simulink model "traj_gene_data"  (R2018b)
settings: Solver=ode4  StartTime=0.0  StopTime=floor(cmd(end,1))  FixedStep=dt_solve  RelTol=1e-3
StopFcn:
  | for k=2:size(imu_delta,1)
  | imu_delta(k-1,2:7) = imu_delta(k,2:7)-imu_delta(k-1,2:7);
  | end
  | imu_delta(1:end-1,1) = imu_delta(2:end,1);
  | imu_delta(end,:) = [];
  | clearvars k
  | save([path,'/traj.mat'], 'traj_m','imu_rate','imu_delta');
values from neighbouring files (symbols this model uses):
  cmd = zeros(1,6)    [traj_design.m]
undefined symbols (not defined in the file or in its folder): data, Earth, Pv, WGS84
libraries: aerolibgravity2 x2, aerolibutil x2, sharedtransform x2, aerolib6dof2 x1, aerolibconvert2 x1
settings Model: Creator=longt  LastModifiedBy=longt
settings DataIOCC: SaveOutput=off  SignalLogging=off  DSMLogging=off  SaveTime=off

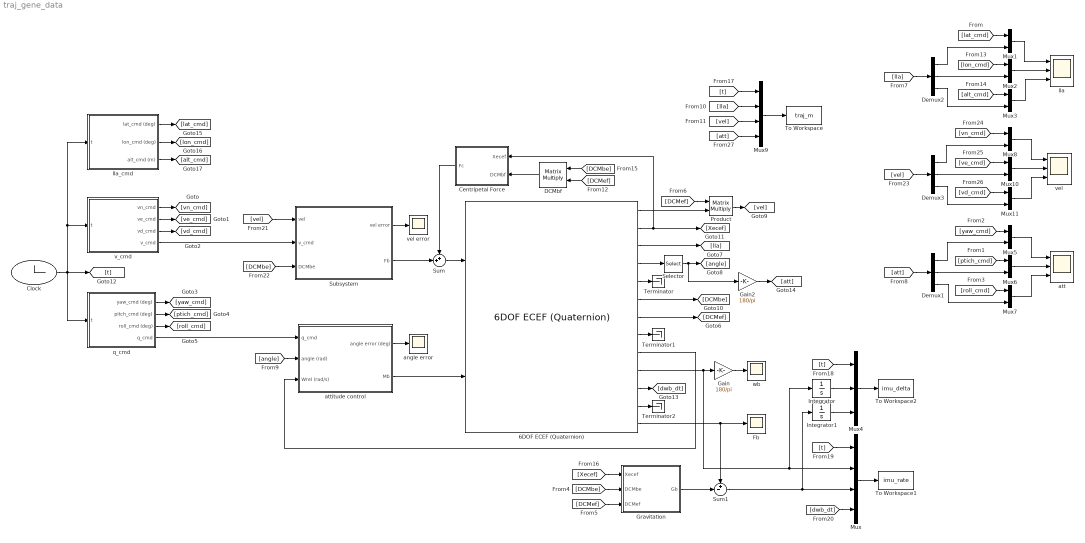
== system traj_gene_data ==
  6DOF ECEF (Quaternion) : aerolib6dof2/6DOF ECEF (Quaternion)  units=Metric (MKS)  mtype=Fixed  xg_0=pos0  Vm_0=[0 0 0]  eul_0=att0  pm_0=[0 0 0]  mass_0=1.0  mass_e=0.5  mass_f=2.0  inertia=eye(3)  inertia_e=eye(3)  inertia_f=2*eye(3)  vre_flag=on  abi_flag=on  ptype=Earth (WGS84)  R=6378137  F=1/298.257223563  w_E=7292115e-11  angle_in=Internal  LG0=0  quat_statename=''  pm_statename=''  Vm_statename=''  posECEF_statename=''  posECI_statename=''  LG_statename=''  mass_statename=''
      settings: SourceProductName=Aerospace Blockset  SourceProductBaseCode=AE
  Centripetal Force : Subsystem
  Clock : Clock
  DCMbf : Product  Multiplication=Matrix(*)
  Demux1 : Demux  Outputs=3
  Demux2 : Demux  Outputs=3
  Demux3 : Demux  Outputs=3
  Fb : Scope
  Gain : Gain  Gain=180/pi
  Gain2 : Gain  Gain=180/pi
  Gravitation : Subsystem
  Integrator : Integrator
  Integrator1 : Integrator
  Mux : Mux
  Mux{1..3,5..8,10..11} (9 alike) : Mux  Inputs=2
  Mux4 : Mux  Inputs=3
  Mux9 : Mux
  Product : Product  Multiplication=Matrix(*)
  Selector : Selector  InputPortWidth=3  IndexOptions=Index vector (dialog)  Indices=[3 2 1]  OutputSizes=1
  Subsystem : Subsystem
  Sum : Sum  Inputs=++|
  Sum1 : Sum  Inputs=+-|
  Terminator : Terminator
  Terminator1 : Terminator
  Terminator2 : Terminator
  To Workspace : ToWorkspace  VariableName=traj_m  SampleTime=-1
      settings: Decimation=dt_traj/dt_solve
  To Workspace1 : ToWorkspace  VariableName=imu_rate  SampleTime=-1
      settings: Decimation=dt_imu_rate/dt_solve
  To Workspace2 : ToWorkspace  VariableName=imu_delta  SampleTime=-1
      settings: Decimation=dt_imu_delta/dt_solve
  angle error : Scope
  att : Scope  NumInputPorts=3
  attitude control : Subsystem
  lla : Scope  NumInputPorts=3
  lla_cmd : Subsystem
  q_cmd : Subsystem
  v_cmd : Subsystem
  vel : Scope  NumInputPorts=3
  vel error : Scope
  wb : Scope
  wires:
  Sum/1 -> 6DOF ECEF (Quaternion)/1
  6DOF ECEF (Quaternion)/2 -> [Xecef], Centripetal Force/1(Xecef)
  6DOF ECEF (Quaternion)/1 -> Product/2
  6DOF ECEF (Quaternion)/7 -> [DCMef]
  DCMbf/1 -> Centripetal Force/2(DCMbf)
  Mux7/1 -> att/3
  Mux6/1 -> att/2
  Mux5/1 -> att/1
  [roll_cmd] -> Mux7/1
  Demux1/3 -> Mux7/2
  Demux1/2 -> Mux6/2
  [yaw_cmd] -> Mux5/1
  6DOF ECEF (Quaternion)/5 -> Terminator/1
  6DOF ECEF (Quaternion)/8 -> Terminator1/1
  6DOF ECEF (Quaternion)/12 -> Terminator2/1
  6DOF ECEF (Quaternion)/10 -> Integrator/1, Mux/2, Gain/1
  6DOF ECEF (Quaternion)/13 -> Sum1/1, Fb/1
  [DCMef] -> Product/1
  Product/1 -> [vel]
  6DOF ECEF (Quaternion)/9 -> attitude control/3(Wrel (rad/s))
  attitude control/1(angle error (deg)) -> angle error/1
  attitude control/2(Mb) -> 6DOF ECEF (Quaternion)/2
  Subsystem/1(vel error) -> vel error/1
  Subsystem/2(Fb) -> Sum/2
  6DOF ECEF (Quaternion)/3 -> [lla]
  Gain/1 -> wb/1
  [angle] -> attitude control/2(angle (rad))
  6DOF ECEF (Quaternion)/4 -> Selector/1
  Mux9/1 -> To Workspace/1
  v_cmd/1(vn_cmd) -> [vn_cmd]
  v_cmd/4(v_cmd) -> Subsystem/2(v_cmd)
  q_cmd/4(q_cmd) -> attitude control/1(q_cmd)
  v_cmd/2(ve_cmd) -> [ve_cmd]
  v_cmd/3(vd_cmd) -> [vd_cmd]
  q_cmd/1(yaw_cmd (deg)) -> [yaw_cmd]
  q_cmd/2(pitch_cmd (deg)) -> [ptich_cmd]
  q_cmd/3(roll_cmd (deg)) -> [roll_cmd]
  Demux2/1 -> Mux1/2
  [lla] -> Demux2/1
  [lat_cmd] -> Mux1/1
  Demux2/2 -> Mux2/2
  [lon_cmd] -> Mux2/1
  Demux2/3 -> Mux3/2
  [alt_cmd] -> Mux3/1
  Mux1/1 -> lla/1
  Mux2/1 -> lla/2
  Mux3/1 -> lla/3
  [ptich_cmd] -> Mux6/1
  6DOF ECEF (Quaternion)/6 -> [DCMbe]
  [DCMbe] -> Gravitation/2(DCMbe)
  [DCMef] -> Gravitation/3(DCMef)
  [DCMef] -> DCMbf/2
  [DCMbe] -> DCMbf/1
  Centripetal Force/1(Fc) -> Sum/1
  [Xecef] -> Gravitation/1(Xecef)
  Mux/1 -> To Workspace1/1
  Mux4/1 -> To Workspace2/1
  [vel] -> Mux9/3
  [lla] -> Mux9/2
  [t] -> Mux9/1
  Integrator/1 -> Mux4/2
  Integrator1/1 -> Mux4/3
  [t] -> Mux4/1
  Demux1/1 -> Mux5/2
  [t] -> Mux/1
  Gravitation/1(Gb) -> Sum1/2
  Sum1/1 -> Integrator1/1, Mux/3
  6DOF ECEF (Quaternion)/11 -> [dwb_dt]
  [dwb_dt] -> Mux/4
  [vel] -> Subsystem/1(vel)
  [DCMbe] -> Subsystem/3(DCMbe)
  [vel] -> Demux3/1
  Mux8/1 -> vel/1
  Mux10/1 -> vel/2
  Mux11/1 -> vel/3
  [vn_cmd] -> Mux8/1
  [ve_cmd] -> Mux10/1
  [vd_cmd] -> Mux11/1
  Demux3/2 -> Mux10/2
  Demux3/1 -> Mux8/2
  Demux3/3 -> Mux11/2
  Gain2/1 -> [att]
  Selector/1 -> [angle], Gain2/1
  [att] -> Demux1/1
  [att] -> Mux9/4
  lla_cmd/2(lon_cmd (deg)) -> [lon_cmd]
  lla_cmd/1(lat_cmd (deg)) -> [lat_cmd]
  lla_cmd/3(alt_cmd (m)) -> [alt_cmd]
  Clock/1 -> q_cmd/1(t), lla_cmd/1(t), v_cmd/1(t), [t]

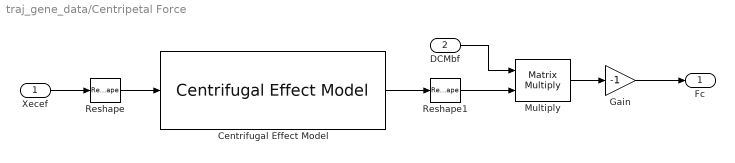
== system traj_gene_data/Centripetal Force ==
  Xecef : Inport
  DCMbf : Inport  Port=2
  Centrifugal Effect Model : aerolibgravity2/Centrifugal Effect Model  ptype=Earth  omega=7.2921150e-05  rate_loc=off
      settings: SourceProductName=Aerospace Blockset  SourceProductBaseCode=AE
  Gain : Gain  Gain=-1
  Multiply : Product  Multiplication=Matrix(*)
  Reshape : Reshape
  Reshape1 : Reshape
  Fc : Outport
  wires:
  Centrifugal Effect Model/1 -> Reshape1/1
  Reshape1/1 -> Multiply/2
  Reshape/1 -> Centrifugal Effect Model/1
  Multiply/1 -> Gain/1
  Xecef/1 -> Reshape/1
  Gain/1 -> Fc/1
  DCMbf/1 -> Multiply/1

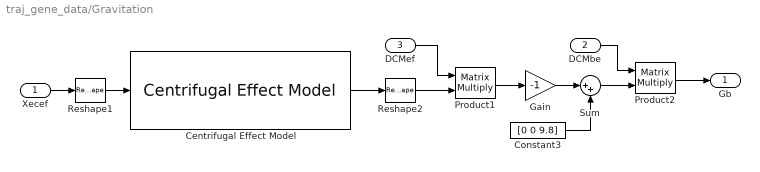
== system traj_gene_data/Gravitation ==
  Xecef : Inport
  DCMbe : Inport  Port=2
  DCMef : Inport  Port=3
  Centrifugal Effect Model : aerolibgravity2/Centrifugal Effect Model  ptype=Earth  omega=7.2921150e-05  rate_loc=off
      settings: SourceProductName=Aerospace Blockset  SourceProductBaseCode=AE
  Constant3 : Constant  Value=[0 0 9.8]
  Gain : Gain  Gain=-1
  Product1 : Product  Multiplication=Matrix(*)
  Product2 : Product  Multiplication=Matrix(*)
  Reshape1 : Reshape
  Reshape2 : Reshape
  Sum : Sum  Inputs=|++
  Gb : Outport
  wires:
  Gain/1 -> Sum/1
  Sum/1 -> Product2/2
  Product1/1 -> Gain/1
  DCMef/1 -> Product1/1
  Xecef/1 -> Reshape1/1
  DCMbe/1 -> Product2/1
  Centrifugal Effect Model/1 -> Reshape2/1
  Reshape2/1 -> Product1/2
  Reshape1/1 -> Centrifugal Effect Model/1
  Product2/1 -> Gb/1
  Constant3/1 -> Sum/2

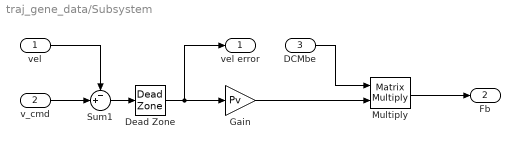
== system traj_gene_data/Subsystem ==
  vel : Inport
  v_cmd : Inport  Port=2
  DCMbe : Inport  Port=3
  Dead Zone : DeadZone  LowerValue=-0.02  UpperValue=0.02  SaturateOnIntegerOverflow=on
  Gain : Gain  Gain=Pv
  Multiply : Product  Multiplication=Matrix(*)
  Sum1 : Sum  Inputs=-+|
  vel error : Outport
  Fb : Outport  Port=2
  wires:
  Gain/1 -> Multiply/2
  Sum1/1 -> Dead Zone/1
  vel/1 -> Sum1/1
  Multiply/1 -> Fb/1
  v_cmd/1 -> Sum1/2
  DCMbe/1 -> Multiply/1
  Dead Zone/1 -> vel error/1, Gain/1

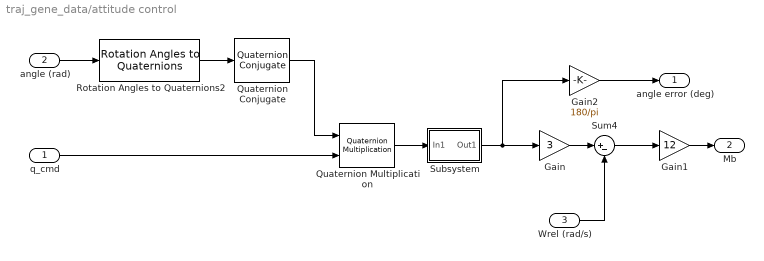
== system traj_gene_data/attitude control ==
  q_cmd : Inport
  angle (rad) : Inport  Port=2
  Wrel (rad/s) : Inport  Port=3
  Gain : Gain  Gain=3
  Gain1 : Gain  Gain=12
  Gain2 : Gain  Gain=180/pi
  Quaternion Conjugate : aerolibutil/Quaternion Conjugate
      settings: SourceProductName=Aerospace Blockset  SourceProductBaseCode=AE
  Quaternion Multiplication : aerolibutil/Quaternion Multiplication
  Rotation Angles to Quaternions2 : sharedtransform/Rotation Angles to Quaternions  rotationOrder=ZYX  aMode=aMode
      settings: SourceProductName=Aerospace Blockset  SourceProductBaseCode=AE
  Subsystem : Subsystem
  Sum4 : Sum  Inputs=|+-
  angle error (deg) : Outport
  Mb : Outport  Port=2
  wires:
  Rotation Angles to Quaternions2/1 -> Quaternion Conjugate/1
  Quaternion Multiplication/1 -> Subsystem/1(In1)
  Quaternion Conjugate/1 -> Quaternion Multiplication/1
  q_cmd/1 -> Quaternion Multiplication/2
  angle (rad)/1 -> Rotation Angles to Quaternions2/1
  Gain2/1 -> angle error (deg)/1
  Wrel (rad/s)/1 -> Sum4/2
  Gain/1 -> Sum4/1
  Gain1/1 -> Mb/1
  Sum4/1 -> Gain1/1
  Subsystem/1(Out1) -> Gain2/1, Gain/1

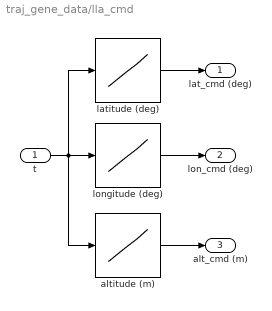
== system traj_gene_data/lla_cmd ==
  t : Inport
  altitude (m) : Lookup_n-D  NumberOfTableDimensions=1  BreakpointsForDimension1=data(:,1)  Table=data(:,4)  InterpMethod=Cubic spline  ExtrapMethod=Clip  InternalRulePriority=Speed  RndMeth=Simplest  InputSameDT=on
  latitude (deg) : Lookup_n-D  NumberOfTableDimensions=1  BreakpointsForDimension1=data(:,1)  Table=data(:,2)  InterpMethod=Cubic spline  ExtrapMethod=Clip  InternalRulePriority=Speed  RndMeth=Simplest  InputSameDT=on
  longitude (deg) : Lookup_n-D  NumberOfTableDimensions=1  BreakpointsForDimension1=data(:,1)  Table=data(:,3)  InterpMethod=Cubic spline  ExtrapMethod=Clip  InternalRulePriority=Speed  RndMeth=Simplest  InputSameDT=on
  lat_cmd (deg) : Outport
  lon_cmd (deg) : Outport  Port=2
  alt_cmd (m) : Outport  Port=3
  wires:
  t/1 -> latitude (deg)/1, altitude (m)/1, longitude (deg)/1
  latitude (deg)/1 -> lat_cmd (deg)/1
  longitude (deg)/1 -> lon_cmd (deg)/1
  altitude (m)/1 -> alt_cmd (m)/1

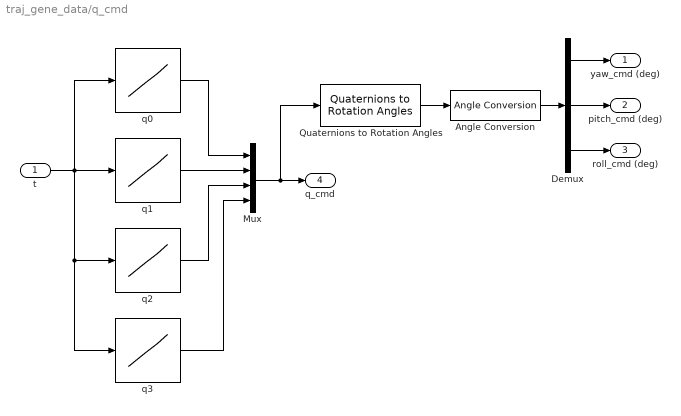
== system traj_gene_data/q_cmd ==
  t : Inport
  Angle Conversion : aerolibconvert2/Angle Conversion  IU=rad  OU=deg
  Demux : Demux  Outputs=3
  Mux : Mux
  Quaternions to Rotation Angles : sharedtransform/Quaternions to Rotation Angles  rotationOrder=ZYX  aMode=aMode
      settings: SourceProductBaseCode=AE
  q0 : Lookup_n-D  NumberOfTableDimensions=1  BreakpointsForDimension1=cmd(:,1)  Table=cmd(:,5)  InterpMethod=Cubic spline  ExtrapMethod=Clip  InternalRulePriority=Speed  RndMeth=Simplest  InputSameDT=on
  q1 : Lookup_n-D  NumberOfTableDimensions=1  BreakpointsForDimension1=cmd(:,1)  Table=cmd(:,6)  InterpMethod=Cubic spline  ExtrapMethod=Clip  InternalRulePriority=Speed  RndMeth=Simplest  InputSameDT=on
  q2 : Lookup_n-D  NumberOfTableDimensions=1  BreakpointsForDimension1=cmd(:,1)  Table=cmd(:,7)  InterpMethod=Cubic spline  ExtrapMethod=Clip  InternalRulePriority=Speed  RndMeth=Simplest  InputSameDT=on
  q3 : Lookup_n-D  NumberOfTableDimensions=1  BreakpointsForDimension1=cmd(:,1)  Table=cmd(:,8)  InterpMethod=Cubic spline  ExtrapMethod=Clip  InternalRulePriority=Speed  RndMeth=Simplest  InputSameDT=on
  yaw_cmd (deg) : Outport
  pitch_cmd (deg) : Outport  Port=2
  roll_cmd (deg) : Outport  Port=3
  q_cmd : Outport  Port=4
  wires:
  t/1 -> q0/1, q2/1, q3/1, q1/1
  q1/1 -> Mux/2
  q0/1 -> Mux/1
  q2/1 -> Mux/3
  q3/1 -> Mux/4
  Mux/1 -> q_cmd/1, Quaternions to Rotation Angles/1
  Quaternions to Rotation Angles/1 -> Angle Conversion/1
  Angle Conversion/1 -> Demux/1
  Demux/1 -> yaw_cmd (deg)/1
  Demux/2 -> pitch_cmd (deg)/1
  Demux/3 -> roll_cmd (deg)/1

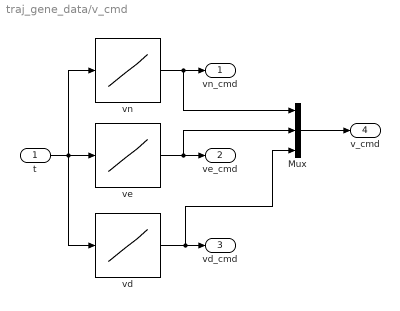
== system traj_gene_data/v_cmd ==
  t : Inport
  Mux : Mux  Inputs=3
  vd : Lookup_n-D  NumberOfTableDimensions=1  BreakpointsForDimension1=cmd(:,1)  Table=cmd(:,4)  InterpMethod=Cubic spline  ExtrapMethod=Clip  InternalRulePriority=Speed  RndMeth=Simplest  InputSameDT=on
  ve : Lookup_n-D  NumberOfTableDimensions=1  BreakpointsForDimension1=cmd(:,1)  Table=cmd(:,3)  InterpMethod=Cubic spline  ExtrapMethod=Clip  InternalRulePriority=Speed  RndMeth=Simplest  InputSameDT=on
  vn : Lookup_n-D  NumberOfTableDimensions=1  BreakpointsForDimension1=cmd(:,1)  Table=cmd(:,2)  InterpMethod=Cubic spline  ExtrapMethod=Clip  InternalRulePriority=Speed  RndMeth=Simplest  InputSameDT=on
  vn_cmd : Outport
  ve_cmd : Outport  Port=2
  vd_cmd : Outport  Port=3
  v_cmd : Outport  Port=4
  wires:
  t/1 -> vn/1, vd/1, ve/1
  Mux/1 -> v_cmd/1
  vn/1 -> Mux/1, vn_cmd/1
  ve/1 -> Mux/2, ve_cmd/1
  vd/1 -> Mux/3, vd_cmd/1

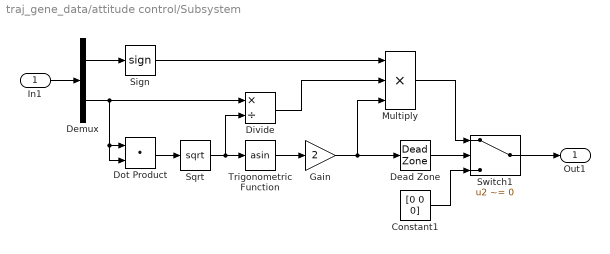
== system traj_gene_data/attitude control/Subsystem ==
  In1 : Inport
  Constant1 : Constant  Value=[0 0 0]
  Dead Zone : DeadZone  LowerValue=-0.01/180*pi  UpperValue=0.01/180*pi  SaturateOnIntegerOverflow=on
  Demux : Demux  Outputs=[1 3]
  Divide : Product  Inputs=*/
  Dot Product : DotProduct  InputSameDT=on  OutDataTypeStr=Inherit: Inherit via internal rule
  Gain : Gain  Gain=2
  Multiply : Product  Inputs=3
  Sign : Signum
  Sqrt : Sqrt  SaturateOnIntegerOverflow=on
  Switch1 : Switch  Criteria=u2 ~= 0
  Trigonometric Function : Trigonometry  Operator=asin
  Out1 : Outport
  wires:
  In1/1 -> Demux/1
  Trigonometric Function/1 -> Gain/1
  Constant1/1 -> Switch1/3
  Switch1/1 -> Out1/1
  Multiply/1 -> Switch1/1
  Sqrt/1 -> Trigonometric Function/1, Divide/2
  Dot Product/1 -> Sqrt/1
  Demux/2 -> Dot Product/2, Dot Product/1, Divide/1
  Demux/1 -> Sign/1
  Divide/1 -> Multiply/2
  Gain/1 -> Dead Zone/1, Multiply/3
  Sign/1 -> Multiply/1
  Dead Zone/1 -> Switch1/2
